simulink model "MyModel"  (R2017a)
settings: Solver=VariableStepAuto  StartTime=0.0  StopTime=10.0  RelTol=1e-3
InitFcn:
  | init
values from neighbouring files (symbols this model uses):
  a = 2    [init.m]
  b = 3    [init.m]
  c = 4    [init.m]
settings Model: Creator=ptracton  LastModifiedBy=ptracton

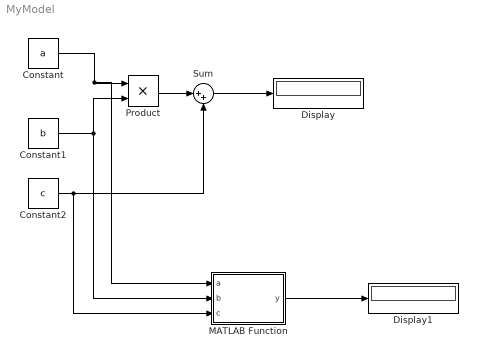
== system MyModel ==
  Constant : Constant  Value=a
  Constant1 : Constant  Value=b
  Constant2 : Constant  Value=c
  Display : Display
  Display1 : Display
  MATLAB Function : MATLAB Function  TreatAsAtomicUnit=on
  Product : Product
  Sum : Sum  Inputs=|++
  wires:
  Constant/1 -> MATLAB Function/1(a), Product/1
  Constant1/1 -> MATLAB Function/2(b), Product/2
  Product/1 -> Sum/1
  Constant2/1 -> MATLAB Function/3(c), Sum/2
  Sum/1 -> Display/1
  MATLAB Function/1(y) -> Display1/1

== matlab function MyModel/MATLAB Function ==
  data: a input; y output; b input; c input
function y = fcn(a,b,c)

y = (a*b)+c;
